simulink model "ALL_JP360_DBW_V6_5_1103"  (R2022a)
settings: Solver=FixedStepAuto  StartTime=0.0  StopTime=inf  FixedStep=0.01  RelTol=1e-3  EnableMultiTasking=on
model workspace (MAT data in the model file):
  g = 9.8
undefined symbols (not defined in the file or in its folder): canChannel, delta_v_p, IPM_Line_C0, IPM_Line_C1, IPM_Line_C2, IPM_Line_C3, M, M_p, MRR_ObjDistX, MRR_ObjDistY, MRR_ObjFusionCamID, MRR_ObjFusionSig, MRR_ObjID, MRR_ObjRelVelX, MRR_ObjRelVelY, MRR_ObjType, MRR_ObjUpdFlg, none, obj_vaild, untracktime, V, videoinput
libraries: canfdmsglib x230, canfdlib x76, slpidlib x24, simulink x18, dspstat3 x14, ctrlSharedLib x1, simulink_extras x1, imaqlib x1, realtime_pacer_lib x1, dspvision x1, visionsinks x1
(part 8 of 55)

== system ALL_JP360_DBW_V6_5_1103/MsgToCAN/CCAN_ADCU_MsgFromCAN ==
  ACC_Torque_Request : Inport
  ACC_Torque_Request_Status : Inport  Port=2
  ACC_TgtAx : Inport  Port=3
  ACC_BrakePreferred : Inport  Port=4
  ACC_StandstillReq : Inport  Port=5
  ACC_Status : Inport  Port=6
  setvspped : Inport  Port=7
  ACC_TimeGapSet : Inport  Port=8
  ACC_EngineStartstop : Inport  Port=9
  IPM_LaneAssit_Status : Inport  Port=10
  IPM_LaneAssit_TorqueReq : Inport  Port=11
  IPM_LaneAssit_TorqueReqStatus : Inport  Port=12
  Obj_Speed : Inport  Port=13
  ACC_ObjDetected : Inport  Port=14
  MRR_L_Obj_0x_class : Inport  Port=15
  MRR_L_Object_dx : Inport  Port=16
  MRR_L_Object_dy : Inport  Port=17
  MRR_LeftTargetDetection : Inport  Port=18
  MRR_R_Obj_0x_class : Inport  Port=19
  MRR_R_Object_dx : Inport  Port=20
  MRR_R_Object_dy : Inport  Port=21
  MRR_RightTargetDetection : Inport  Port=22
  MRR_F_Object_dx : Inport  Port=23
  MRR_F_Object_dy : Inport  Port=24
  MRR_F_Obj_0x_class : Inport  Port=25
  640 : Inport  Port=26
  641 : Inport  Port=27
  642 : Inport  Port=28
  643 : Inport  Port=29
  ACC_DriveOff : Inport  Port=30
  Add : Sum  Inputs=+-
  Bus Selector : BusSelector  OutputSignals=IPM_Line01_Existence_Probability,IPM_Line01_ColorClass,IPM_Line01_Type
  Bus Selector1 : BusSelector  OutputSignals=IPM_Line02_Existence_Probability,IPM_Line02_Type,IPM_Line02_ColorClass
  CCAN_ADCU_ADCU_0x538 : Subsystem  Commented=on  TreatAsAtomicUnit=on
  CCAN_ADCU_ADCU_CanTSyn_0x570 : Subsystem  Commented=on  TreatAsAtomicUnit=on
  CCAN_ADCU_ADCU_DiagResp : Subsystem  Commented=on  TreatAsAtomicUnit=on
  CCAN_ADCU_IPM_0x245 : Subsystem  TreatAsAtomicUnit=on  SystemSampleTime=0.02
  CCAN_ADCU_IPM_0x247 : Subsystem  Commented=on  TreatAsAtomicUnit=on
  CCAN_ADCU_IPM_LeftLine_0x278 : Subsystem  TreatAsAtomicUnit=on
  CCAN_ADCU_IPM_LeftLine_0x280 : Subsystem  TreatAsAtomicUnit=on
  CCAN_ADCU_IPM_RightLine_0x490 : Subsystem  TreatAsAtomicUnit=on
  CCAN_ADCU_IPM_RightLine_0x491 : Subsystem  TreatAsAtomicUnit=on
  CCAN_ADCU_IPM_VLC_0x293 : Subsystem  TreatAsAtomicUnit=on  SystemSampleTime=0.02
  CCAN_ADCU_MRR_0x238 : Subsystem  TreatAsAtomicUnit=on  SystemSampleTime=0.02
  CCAN_ADCU_MRR_0x239 : Subsystem  TreatAsAtomicUnit=on  SystemSampleTime=0.02
  CCAN_ADCU_MRR_0x246 : Subsystem  TreatAsAtomicUnit=on  SystemSampleTime=0.02
  CCAN_ADCU_MRR_FRObj_0x279 : Subsystem  TreatAsAtomicUnit=on
  CCAN_ADCU_MRR_LRObj_0x480 : Subsystem  TreatAsAtomicUnit=on
  CCAN_ADCU_TIMESYNC_analy_620 : Subsystem  Commented=on  TreatAsAtomicUnit=on
  Constant : Constant  OutDataTypeStr=int8
  Constant1 : Constant  Value=0  OutDataTypeStr=boolean
  Constant5 : Constant  Value=4  OutDataTypeStr=int8
  Constant6 : Constant  Value=2  OutDataTypeStr=int8
  Constant7 : Constant  OutDataTypeStr=int8
  Product : Product
  Product1 : Product
  Switch1 : Switch  Criteria=u2 > Threshold  Threshold=0.7  SaturateOnIntegerOverflow=off  InputSameDT=off
  Switch2 : Switch  Criteria=u2 > Threshold  Threshold=0.7  SaturateOnIntegerOverflow=off  InputSameDT=off
  Switch3 : Switch  Criteria=u2 ~= 0  SaturateOnIntegerOverflow=off  InputSameDT=off
  CCAN_ADCU_ADCU_0x538FromOutData : Outport  OutDataTypeStr=Bus:CCAN_ADCU_ADCU_0x538
  CCAN_ADCU_ADCU_CanTSyn_0x570FromOutData : Outport  Port=2  OutDataTypeStr=Bus:CCAN_ADCU_ADCU_CanTSyn_0x570
  CCAN_ADCU_ADCU_DiagRespFromOutData : Outport  Port=3  OutDataTypeStr=Bus:CCAN_ADCU_ADCU_DiagResp
  CCAN_ADCU_IPM_0x245FromOutData : Outport  Port=4  OutDataTypeStr=Bus:CCAN_ADCU_IPM_0x245
  CCAN_ADCU_IPM_0x247FromOutData : Outport  Port=5  OutDataTypeStr=Bus:CCAN_ADCU_IPM_0x247
  CCAN_ADCU_IPM_LeftLine_0x278FromOutData : Outport  Port=6  OutDataTypeStr=Bus:CCAN_ADCU_IPM_LeftLine_0x278
  CCAN_ADCU_IPM_LeftLine_0x280FromOutData : Outport  Port=7  OutDataTypeStr=Bus:CCAN_ADCU_IPM_LeftLine_0x280
  CCAN_ADCU_IPM_RightLine_0x490FromOutData : Outport  Port=8  OutDataTypeStr=Bus:CCAN_ADCU_IPM_RightLine_0x490
  CCAN_ADCU_IPM_RightLine_0x491FromOutData : Outport  Port=9  OutDataTypeStr=Bus:CCAN_ADCU_IPM_RightLine_0x491
  CCAN_ADCU_IPM_VLC_0x293FromOutData : Outport  Port=10  OutDataTypeStr=Bus:CCAN_ADCU_IPM_VLC_0x293
  CCAN_ADCU_MRR_0x238FromOutData : Outport  Port=11  OutDataTypeStr=Bus:CCAN_ADCU_MRR_0x238
  CCAN_ADCU_MRR_0x239FromOutData : Outport  Port=12  OutDataTypeStr=Bus:CCAN_ADCU_MRR_0x239
  CCAN_ADCU_MRR_0x246FromOutData : Outport  Port=13  OutDataTypeStr=Bus:CCAN_ADCU_MRR_0x246
  CCAN_ADCU_MRR_FRObj_0x279FromOutData : Outport  Port=14  OutDataTypeStr=Bus:CCAN_ADCU_MRR_FRObj_0x279
  CCAN_ADCU_MRR_LRObj_0x480FromOutData : Outport  Port=15  OutDataTypeStr=Bus:CCAN_ADCU_MRR_LRObj_0x480
  CCAN_ADCU_TIMESYNC_analy_620FromOutData : Outport  Port=16  OutDataTypeStr=Bus:CCAN_ADCU_TIMESYNC_analy_620
  wires:
  CCAN_ADCU_ADCU_0x538/1(CCAN_ADCU_ADCU_0x538FromOutData) -> CCAN_ADCU_ADCU_0x538FromOutData/1
  CCAN_ADCU_ADCU_CanTSyn_0x570/1(CCAN_ADCU_ADCU_CanTSyn_0x570FromOutData) -> CCAN_ADCU_ADCU_CanTSyn_0x570FromOutData/1
  CCAN_ADCU_ADCU_DiagResp/1(CCAN_ADCU_ADCU_DiagRespFromOutData) -> CCAN_ADCU_ADCU_DiagRespFromOutData/1
  CCAN_ADCU_IPM_0x245/1(CCAN_ADCU_IPM_0x245FromOutData) -> CCAN_ADCU_IPM_0x245FromOutData/1
  CCAN_ADCU_IPM_0x247/1(CCAN_ADCU_IPM_0x247FromOutData) -> CCAN_ADCU_IPM_0x247FromOutData/1
  CCAN_ADCU_IPM_LeftLine_0x278/1(CCAN_ADCU_IPM_LeftLine_0x278FromOutData) -> CCAN_ADCU_IPM_LeftLine_0x278FromOutData/1
  CCAN_ADCU_IPM_LeftLine_0x280/1(CCAN_ADCU_IPM_LeftLine_0x280FromOutData) -> CCAN_ADCU_IPM_LeftLine_0x280FromOutData/1
  CCAN_ADCU_IPM_RightLine_0x490/1(CCAN_ADCU_IPM_RightLine_0x490FromOutData) -> CCAN_ADCU_IPM_RightLine_0x490FromOutData/1
  CCAN_ADCU_IPM_RightLine_0x491/1(CCAN_ADCU_IPM_RightLine_0x491FromOutData) -> CCAN_ADCU_IPM_RightLine_0x491FromOutData/1
  CCAN_ADCU_IPM_VLC_0x293/1(CCAN_ADCU_IPM_VLC_0x293FromOutData) -> CCAN_ADCU_IPM_VLC_0x293FromOutData/1
  CCAN_ADCU_MRR_0x238/1(CCAN_ADCU_MRR_0x238FromOutData) -> CCAN_ADCU_MRR_0x238FromOutData/1
  CCAN_ADCU_MRR_0x239/1(CCAN_ADCU_MRR_0x239FromOutData) -> CCAN_ADCU_MRR_0x239FromOutData/1
  CCAN_ADCU_MRR_0x246/1(CCAN_ADCU_MRR_0x246FromOutData) -> CCAN_ADCU_MRR_0x246FromOutData/1
  CCAN_ADCU_MRR_FRObj_0x279/1(CCAN_ADCU_MRR_FRObj_0x279FromOutData) -> CCAN_ADCU_MRR_FRObj_0x279FromOutData/1
  CCAN_ADCU_MRR_LRObj_0x480/1(CCAN_ADCU_MRR_LRObj_0x480FromOutData) -> CCAN_ADCU_MRR_LRObj_0x480FromOutData/1
  CCAN_ADCU_TIMESYNC_analy_620/1(CCAN_ADCU_TIMESYNC_analy_620FromOutData) -> CCAN_ADCU_TIMESYNC_analy_620FromOutData/1
  ACC_Torque_Request/1 -> CCAN_ADCU_IPM_VLC_0x293/1(ACC_Torque_Request)
  ACC_Torque_Request_Status/1 -> CCAN_ADCU_IPM_VLC_0x293/2(ACC_Torque_Request_Status)
  ACC_TgtAx/1 -> CCAN_ADCU_MRR_0x238/1(ACC_TgtAx)
  ACC_StandstillReq/1 -> CCAN_ADCU_MRR_0x239/3(ACC_StandstillReq)
  ACC_BrakePreferred/1 -> CCAN_ADCU_MRR_0x239/1(ACC_BrakePreferred)
  ACC_Status/1 -> CCAN_ADCU_MRR_0x246/1(ACC_Status), CCAN_ADCU_MRR_0x239/2(ACC_Status)
  ACC_EngineStartstop/1 -> CCAN_ADCU_MRR_0x246/4(ACC_EngineStartstop)
  ACC_TimeGapSet/1 -> CCAN_ADCU_MRR_0x246/3(ACC_TimeGapSet)
  setvspped/1 -> CCAN_ADCU_MRR_0x246/2(setvspped)
  IPM_LaneAssit_TorqueReqStatus/1 -> CCAN_ADCU_IPM_0x245/3(IPM_LaneAssit_TorqueReqStatus)
  IPM_LaneAssit_TorqueReq/1 -> CCAN_ADCU_IPM_0x245/2(IPM_LaneAssit_TorqueReq)
  IPM_LaneAssit_Status/1 -> CCAN_ADCU_IPM_0x245/1(IPM_LaneAssit_Status), [LKAStatus]
  Obj_Speed/1 -> CCAN_ADCU_MRR_0x246/5(Obj_Speed)
  ACC_ObjDetected/1 -> CCAN_ADCU_MRR_0x246/6(ACC_ObjDetected)
  MRR_L_Obj_0x_class/1 -> CCAN_ADCU_MRR_LRObj_0x480/1(MRR_L_Obj_0x_class)
  MRR_L_Object_dx/1 -> CCAN_ADCU_MRR_LRObj_0x480/2(MRR_L_Object_dx)
  MRR_L_Object_dy/1 -> CCAN_ADCU_MRR_LRObj_0x480/3(MRR_L_Object_dy)
  MRR_LeftTargetDetection/1 -> CCAN_ADCU_MRR_LRObj_0x480/4(MRR_LeftTargetDetection)
  MRR_R_Obj_0x_class/1 -> CCAN_ADCU_MRR_LRObj_0x480/5(MRR_R_Obj_0x_class)
  MRR_R_Object_dx/1 -> CCAN_ADCU_MRR_LRObj_0x480/6(MRR_R_Object_dx)
  MRR_R_Object_dy/1 -> CCAN_ADCU_MRR_LRObj_0x480/7(MRR_R_Object_dy)
  MRR_RightTargetDetection/1 -> CCAN_ADCU_MRR_LRObj_0x480/8(MRR_RightTargetDetection)
  MRR_F_Obj_0x_class/1 -> CCAN_ADCU_MRR_FRObj_0x279/3(MRR_F_Obj_0x_class)
  MRR_F_Object_dy/1 -> CCAN_ADCU_MRR_FRObj_0x279/2(MRR_F_Object_dy)
  MRR_F_Object_dx/1 -> CCAN_ADCU_MRR_FRObj_0x279/1(MRR_F_Object_dx)
  643/1 -> CCAN_ADCU_IPM_RightLine_0x491/3(491)
  642/1 -> CCAN_ADCU_IPM_LeftLine_0x280/3(280)
  640/1 -> Bus Selector/1, CCAN_ADCU_IPM_LeftLine_0x278/1(278)
  Bus Selector/2 -> CCAN_ADCU_IPM_LeftLine_0x280/2(In1)  "<IPM_Line01_ColorClass>"
  Bus Selector/3 -> CCAN_ADCU_IPM_LeftLine_0x280/1(In2)  "<IPM_Line01_Type>"
  641/1 -> Bus Selector1/1, CCAN_ADCU_IPM_RightLine_0x490/1(490)
  Bus Selector1/2 -> CCAN_ADCU_IPM_RightLine_0x491/2(In1)  "<IPM_Line02_Type>"
  Bus Selector1/3 -> CCAN_ADCU_IPM_RightLine_0x491/1(In2)  "<IPM_Line02_ColorClass>"
  Bus Selector/1 -> [line01]  "<IPM_Line01_Existence_Probability>"
  Bus Selector1/1 -> [line02]  "<IPM_Line02_Existence_Probability>"
  Product/1 -> CCAN_ADCU_IPM_0x245/4(line01)
  Product1/1 -> CCAN_ADCU_IPM_0x245/5(line02)
  ACC_DriveOff/1 -> CCAN_ADCU_MRR_0x239/4(ACC_DriveOff)
  [line02] -> Switch2/2
  Switch1/1 -> Product/1
  Constant/1 -> Switch2/1, Switch1/1
  Switch2/1 -> Product1/1
  [line01] -> Switch1/2
  Add/1 -> Switch3/2
  Constant7/1 -> Switch3/1
  Constant5/1 -> Add/2
  [LKAStatus] -> Add/1
  Constant6/1 -> Switch3/3
  Constant1/1 -> Switch1/3, Switch2/3
  Switch3/1 -> Product/2, Product1/2

== system ALL_JP360_DBW_V6_5_1103/MsgToCAN/CCAN_ADCU_MsgToCAN ==
  CCAN_ADCU_ADCU_0x538ToInData : Inport  OutDataTypeStr=Bus:CCAN_ADCU_ADCU_0x538
  CCAN_ADCU_ADCU_CanTSyn_0x570ToInData : Inport  Port=2  OutDataTypeStr=Bus:CCAN_ADCU_ADCU_CanTSyn_0x570
  CCAN_ADCU_ADCU_DiagRespToInData : Inport  Port=3  OutDataTypeStr=Bus:CCAN_ADCU_ADCU_DiagResp
  CCAN_ADCU_IPM_0x245ToInData : Inport  Port=4  OutDataTypeStr=Bus:CCAN_ADCU_IPM_0x245
  CCAN_ADCU_IPM_0x247ToInData : Inport  Port=5  OutDataTypeStr=Bus:CCAN_ADCU_IPM_0x247
  CCAN_ADCU_IPM_LeftLine_0x278ToInData : Inport  Port=6  OutDataTypeStr=Bus:CCAN_ADCU_IPM_LeftLine_0x278
  CCAN_ADCU_IPM_LeftLine_0x280ToInData : Inport  Port=7  OutDataTypeStr=Bus:CCAN_ADCU_IPM_LeftLine_0x280
  CCAN_ADCU_IPM_RightLine_0x490ToInData : Inport  Port=8  OutDataTypeStr=Bus:CCAN_ADCU_IPM_RightLine_0x490
  CCAN_ADCU_IPM_RightLine_0x491ToInData : Inport  Port=9  OutDataTypeStr=Bus:CCAN_ADCU_IPM_RightLine_0x491
  CCAN_ADCU_IPM_VLC_0x293ToInData : Inport  Port=10  OutDataTypeStr=Bus:CCAN_ADCU_IPM_VLC_0x293
  CCAN_ADCU_MRR_0x238ToInData : Inport  Port=11  OutDataTypeStr=Bus:CCAN_ADCU_MRR_0x238
  CCAN_ADCU_MRR_0x239ToInData : Inport  Port=12  OutDataTypeStr=Bus:CCAN_ADCU_MRR_0x239
  CCAN_ADCU_MRR_0x246ToInData : Inport  Port=13  OutDataTypeStr=Bus:CCAN_ADCU_MRR_0x246
  CCAN_ADCU_MRR_FRObj_0x279ToInData : Inport  Port=14  OutDataTypeStr=Bus:CCAN_ADCU_MRR_FRObj_0x279
  CCAN_ADCU_MRR_LRObj_0x480ToInData : Inport  Port=15  OutDataTypeStr=Bus:CCAN_ADCU_MRR_LRObj_0x480
  CCAN_ADCU_TIMESYNC_analy_620ToInData : Inport  Port=16  OutDataTypeStr=Bus:CCAN_ADCU_TIMESYNC_analy_620
  CCAN_ADCU_ADCU_0x538 : Subsystem  TreatAsAtomicUnit=on
  CCAN_ADCU_ADCU_CanTSyn_0x570 : Subsystem  TreatAsAtomicUnit=on
  CCAN_ADCU_ADCU_DiagResp : Subsystem  TreatAsAtomicUnit=on
  CCAN_ADCU_IPM_0x245 : Subsystem  TreatAsAtomicUnit=on
  CCAN_ADCU_IPM_0x247 : Subsystem  TreatAsAtomicUnit=on
  CCAN_ADCU_IPM_LeftLine_0x278 : Subsystem  TreatAsAtomicUnit=on
  CCAN_ADCU_IPM_LeftLine_0x280 : Subsystem  TreatAsAtomicUnit=on
  CCAN_ADCU_IPM_RightLine_0x490 : Subsystem  TreatAsAtomicUnit=on
  CCAN_ADCU_IPM_RightLine_0x491 : Subsystem  TreatAsAtomicUnit=on
  CCAN_ADCU_IPM_VLC_0x293 : Subsystem  TreatAsAtomicUnit=on
  CCAN_ADCU_MRR_0x238 : Subsystem  TreatAsAtomicUnit=on
  CCAN_ADCU_MRR_0x239 : Subsystem  TreatAsAtomicUnit=on
  CCAN_ADCU_MRR_0x246 : Subsystem  TreatAsAtomicUnit=on
  CCAN_ADCU_MRR_FRObj_0x279 : Subsystem  TreatAsAtomicUnit=on
  CCAN_ADCU_MRR_LRObj_0x480 : Subsystem  TreatAsAtomicUnit=on
  CCAN_ADCU_TIMESYNC_analy_620 : Subsystem  TreatAsAtomicUnit=on
  CCAN_ADCU_ADCU_0x538ToOutData : Outport  OutDataTypeStr=Bus:CAN_FD_MESSAGE_BUS
  CCAN_ADCU_ADCU_CanTSyn_0x570ToOutData : Outport  Port=2  OutDataTypeStr=Bus:CAN_FD_MESSAGE_BUS
  CCAN_ADCU_ADCU_DiagRespToOutData : Outport  Port=3  OutDataTypeStr=Bus:CAN_FD_MESSAGE_BUS
  CCAN_ADCU_IPM_0x245ToOutData : Outport  Port=4  OutDataTypeStr=Bus:CAN_FD_MESSAGE_BUS
  CCAN_ADCU_IPM_0x247ToOutData : Outport  Port=5  OutDataTypeStr=Bus:CAN_FD_MESSAGE_BUS
  CCAN_ADCU_IPM_LeftLine_0x278ToOutData : Outport  Port=6  OutDataTypeStr=Bus:CAN_FD_MESSAGE_BUS
  CCAN_ADCU_IPM_LeftLine_0x280ToOutData : Outport  Port=7  OutDataTypeStr=Bus:CAN_FD_MESSAGE_BUS
  CCAN_ADCU_IPM_RightLine_0x490ToOutData : Outport  Port=8  OutDataTypeStr=Bus:CAN_FD_MESSAGE_BUS
  CCAN_ADCU_IPM_RightLine_0x491ToOutData : Outport  Port=9  OutDataTypeStr=Bus:CAN_FD_MESSAGE_BUS
  CCAN_ADCU_IPM_VLC_0x293ToOutData : Outport  Port=10  OutDataTypeStr=Bus:CAN_FD_MESSAGE_BUS
  CCAN_ADCU_MRR_0x238ToOutData : Outport  Port=11  OutDataTypeStr=Bus:CAN_FD_MESSAGE_BUS
  CCAN_ADCU_MRR_0x239ToOutData : Outport  Port=12  OutDataTypeStr=Bus:CAN_FD_MESSAGE_BUS
  CCAN_ADCU_MRR_0x246ToOutData : Outport  Port=13  OutDataTypeStr=Bus:CAN_FD_MESSAGE_BUS
  CCAN_ADCU_MRR_FRObj_0x279ToOutData : Outport  Port=14  OutDataTypeStr=Bus:CAN_FD_MESSAGE_BUS
  CCAN_ADCU_MRR_LRObj_0x480ToOutData : Outport  Port=15  OutDataTypeStr=Bus:CAN_FD_MESSAGE_BUS
  CCAN_ADCU_TIMESYNC_analy_620ToOutData : Outport  Port=16  OutDataTypeStr=Bus:CAN_FD_MESSAGE_BUS
  wires:
  CCAN_ADCU_ADCU_0x538ToInData/1 -> CCAN_ADCU_ADCU_0x538/1(CCAN_ADCU_ADCU_0x538ToInData)  "CCAN_ADCU_ADCU_0x538ToInData"
  CCAN_ADCU_ADCU_0x538/1(CCAN_ADCU_ADCU_0x538ToOutData) -> CCAN_ADCU_ADCU_0x538ToOutData/1  "CCAN_ADCU_ADCU_0x538ToOutData"
  CCAN_ADCU_ADCU_CanTSyn_0x570ToInData/1 -> CCAN_ADCU_ADCU_CanTSyn_0x570/1(CCAN_ADCU_ADCU_CanTSyn_0x570ToInData)  "CCAN_ADCU_ADCU_CanTSyn_0x570ToInData"
  CCAN_ADCU_ADCU_CanTSyn_0x570/1(CCAN_ADCU_ADCU_CanTSyn_0x570ToOutData) -> CCAN_ADCU_ADCU_CanTSyn_0x570ToOutData/1  "CCAN_ADCU_ADCU_CanTSyn_0x570ToOutData"
  CCAN_ADCU_ADCU_DiagRespToInData/1 -> CCAN_ADCU_ADCU_DiagResp/1(CCAN_ADCU_ADCU_DiagRespToInData)  "CCAN_ADCU_ADCU_DiagRespToInData"
  CCAN_ADCU_ADCU_DiagResp/1(CCAN_ADCU_ADCU_DiagRespToOutData) -> CCAN_ADCU_ADCU_DiagRespToOutData/1  "CCAN_ADCU_ADCU_DiagRespToOutData"
  CCAN_ADCU_IPM_0x245ToInData/1 -> CCAN_ADCU_IPM_0x245/1(CCAN_ADCU_IPM_0x245ToInData)  "CCAN_ADCU_IPM_0x245ToInData"
  CCAN_ADCU_IPM_0x245/1(CCAN_ADCU_IPM_0x245ToOutData) -> CCAN_ADCU_IPM_0x245ToOutData/1  "CCAN_ADCU_IPM_0x245ToOutData"
  CCAN_ADCU_IPM_0x247ToInData/1 -> CCAN_ADCU_IPM_0x247/1(CCAN_ADCU_IPM_0x247ToInData)  "CCAN_ADCU_IPM_0x247ToInData"
  CCAN_ADCU_IPM_0x247/1(CCAN_ADCU_IPM_0x247ToOutData) -> CCAN_ADCU_IPM_0x247ToOutData/1  "CCAN_ADCU_IPM_0x247ToOutData"
  CCAN_ADCU_IPM_LeftLine_0x278ToInData/1 -> CCAN_ADCU_IPM_LeftLine_0x278/1(CCAN_ADCU_IPM_LeftLine_0x278ToInData)  "CCAN_ADCU_IPM_LeftLine_0x278ToInData"
  CCAN_ADCU_IPM_LeftLine_0x278/1(CCAN_ADCU_IPM_LeftLine_0x278ToOutData) -> CCAN_ADCU_IPM_LeftLine_0x278ToOutData/1  "CCAN_ADCU_IPM_LeftLine_0x278ToOutData"
  CCAN_ADCU_IPM_LeftLine_0x280ToInData/1 -> CCAN_ADCU_IPM_LeftLine_0x280/1(CCAN_ADCU_IPM_LeftLine_0x280ToInData)  "CCAN_ADCU_IPM_LeftLine_0x280ToInData"
  CCAN_ADCU_IPM_LeftLine_0x280/1(CCAN_ADCU_IPM_LeftLine_0x280ToOutData) -> CCAN_ADCU_IPM_LeftLine_0x280ToOutData/1  "CCAN_ADCU_IPM_LeftLine_0x280ToOutData"
  CCAN_ADCU_IPM_RightLine_0x490ToInData/1 -> CCAN_ADCU_IPM_RightLine_0x490/1(CCAN_ADCU_IPM_RightLine_0x490ToInData)  "CCAN_ADCU_IPM_RightLine_0x490ToInData"
  CCAN_ADCU_IPM_RightLine_0x490/1(CCAN_ADCU_IPM_RightLine_0x490ToOutData) -> CCAN_ADCU_IPM_RightLine_0x490ToOutData/1  "CCAN_ADCU_IPM_RightLine_0x490ToOutData"
  CCAN_ADCU_IPM_RightLine_0x491ToInData/1 -> CCAN_ADCU_IPM_RightLine_0x491/1(CCAN_ADCU_IPM_RightLine_0x491ToInData)  "CCAN_ADCU_IPM_RightLine_0x491ToInData"
  CCAN_ADCU_IPM_RightLine_0x491/1(CCAN_ADCU_IPM_RightLine_0x491ToOutData) -> CCAN_ADCU_IPM_RightLine_0x491ToOutData/1  "CCAN_ADCU_IPM_RightLine_0x491ToOutData"
  CCAN_ADCU_IPM_VLC_0x293ToInData/1 -> CCAN_ADCU_IPM_VLC_0x293/1(CCAN_ADCU_IPM_VLC_0x293ToInData)  "CCAN_ADCU_IPM_VLC_0x293ToInData"
  CCAN_ADCU_IPM_VLC_0x293/1(CCAN_ADCU_IPM_VLC_0x293ToOutData) -> CCAN_ADCU_IPM_VLC_0x293ToOutData/1  "CCAN_ADCU_IPM_VLC_0x293ToOutData"
  CCAN_ADCU_MRR_0x238ToInData/1 -> CCAN_ADCU_MRR_0x238/1(CCAN_ADCU_MRR_0x238ToInData)  "CCAN_ADCU_MRR_0x238ToInData"
  CCAN_ADCU_MRR_0x238/1(CCAN_ADCU_MRR_0x238ToOutData) -> CCAN_ADCU_MRR_0x238ToOutData/1  "CCAN_ADCU_MRR_0x238ToOutData"
  CCAN_ADCU_MRR_0x239ToInData/1 -> CCAN_ADCU_MRR_0x239/1(CCAN_ADCU_MRR_0x239ToInData)  "CCAN_ADCU_MRR_0x239ToInData"
  CCAN_ADCU_MRR_0x239/1(CCAN_ADCU_MRR_0x239ToOutData) -> CCAN_ADCU_MRR_0x239ToOutData/1  "CCAN_ADCU_MRR_0x239ToOutData"
  CCAN_ADCU_MRR_0x246ToInData/1 -> CCAN_ADCU_MRR_0x246/1(CCAN_ADCU_MRR_0x246ToInData)  "CCAN_ADCU_MRR_0x246ToInData"
  CCAN_ADCU_MRR_0x246/1(CCAN_ADCU_MRR_0x246ToOutData) -> CCAN_ADCU_MRR_0x246ToOutData/1  "CCAN_ADCU_MRR_0x246ToOutData"
  CCAN_ADCU_MRR_FRObj_0x279ToInData/1 -> CCAN_ADCU_MRR_FRObj_0x279/1(CCAN_ADCU_MRR_FRObj_0x279ToInData)  "CCAN_ADCU_MRR_FRObj_0x279ToInData"
  CCAN_ADCU_MRR_FRObj_0x279/1(CCAN_ADCU_MRR_FRObj_0x279ToOutData) -> CCAN_ADCU_MRR_FRObj_0x279ToOutData/1  "CCAN_ADCU_MRR_FRObj_0x279ToOutData"
  CCAN_ADCU_MRR_LRObj_0x480ToInData/1 -> CCAN_ADCU_MRR_LRObj_0x480/1(CCAN_ADCU_MRR_LRObj_0x480ToInData)  "CCAN_ADCU_MRR_LRObj_0x480ToInData"
  CCAN_ADCU_MRR_LRObj_0x480/1(CCAN_ADCU_MRR_LRObj_0x480ToOutData) -> CCAN_ADCU_MRR_LRObj_0x480ToOutData/1  "CCAN_ADCU_MRR_LRObj_0x480ToOutData"
  CCAN_ADCU_TIMESYNC_analy_620ToInData/1 -> CCAN_ADCU_TIMESYNC_analy_620/1(CCAN_ADCU_TIMESYNC_analy_620ToInData)  "CCAN_ADCU_TIMESYNC_analy_620ToInData"
  CCAN_ADCU_TIMESYNC_analy_620/1(CCAN_ADCU_TIMESYNC_analy_620ToOutData) -> CCAN_ADCU_TIMESYNC_analy_620ToOutData/1  "CCAN_ADCU_TIMESYNC_analy_620ToOutData"

== system ALL_JP360_DBW_V6_5_1103/button/ACCset ==
  note: 0: OFF
      | 1: Passive
      | 2: Stand-By
      | 3: Active-Control
      | 5: Override
      | 6: Standstill
      | 7: Failure
  SWM_ACCSwitch : Inport
  acc_status : Inport  Port=2  OutDataTypeStr=int8
  set_speed_out : Inport  Port=3
  TimeGapSet : Inport  Port=4
  SWM_ACCvSetPlus : Inport  Port=5
  SWM_ACCvSetMinus : Inport  Port=6
  ACC_button : Subsystem
  Chart1 : Stateflow chart  TreatAsAtomicUnit=on
  accsetv4 : Stateflow chart  TreatAsAtomicUnit=on
      settings: RTWSystemCode=Reusable function
  setvspeed : Outport
  TimeGapSetOut : Outport  Port=2
  Out3 : Outport  Port=3
  wires:
  TimeGapSet/1 -> Chart1/Trigger
  SWM_ACCSwitch/1 -> [SWM_ACCSwitch]
  SWM_ACCvSetPlus/1 -> [SWM_ACCvSetPlus]
  SWM_ACCvSetMinus/1 -> [SWM_ACCvSetMinus]
  Chart1/1(TimeGapSet) -> accsetv4/2(speed)
  [accsinp] -> accsetv4/1(accs)
  accsetv4/1(speedout) -> TimeGapSetOut/1
  ACC_button/1(setvspeed) -> setvspeed/1
  acc_status/1 -> ACC_button/1(Input), [accsinp]
  [SWM_ACCvSetMinus] -> ACC_button/4(SWM_ACCvSetMinus)
  [SWM_ACCvSetPlus] -> ACC_button/3(SWM_ACCvSetPlus)
  [SWM_ACCSwitch] -> ACC_button/2(SWM_ACCSwitch)
  ACC_button/2(SWM_ACCSwitchOut) -> Out3/1
  set_speed_out/1 -> ACC_button/5(set_speed_out)

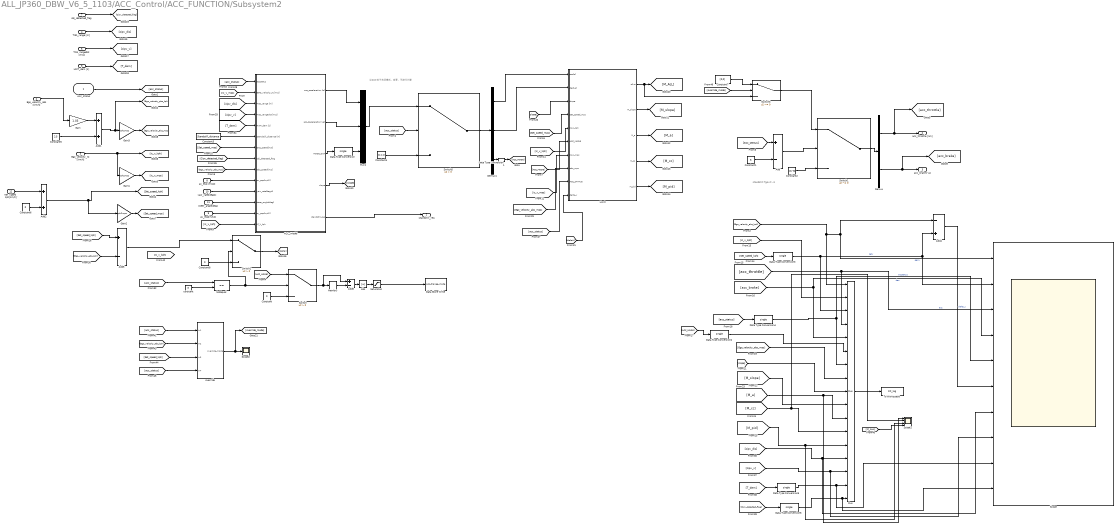
== system ALL_JP360_DBW_V6_5_1103/ACC_Control/ACC_FUNCTION/Subsystem2 ==
  note: standstill
      | TgAx= -3
  note: 当ACC处于关闭模式，发零，不进行计算
  Acc_status : Inport
  Ego_velocity_abs [km/h] : Inport  Port=2
  Ego_velocity_IC [km/h] : Inport  Port=3
  TIS1_range [m] : Inport  Port=4
  TIS1_rangedot [m/s] : Inport  Port=5
  HWT_dem [s] : Inport  Port=6
  obj_detacted_flag : Inport  Port=7
  ax_esp [m/s2] : Inport  Port=8
  ay_esp[m/s2] : Inport  Port=9
  yaw_rate[deg/s] : Inport  Port=10
  steer_angle[deg] : Inport  Port=11
  Set_speed_kph[km/h] : Inport  Port=12
  ACC_model : Subsystem
  Abs : Abs  SaturateOnIntegerOverflow=off
  Add : Sum  Inputs=+-
  Add1 : Sum
  Add2 : Sum
  Add4 : Sum  Inputs=-+
  Add5 : Sum  Inputs=+-
  Add6 : Sum  Inputs=+-
  Constant : Constant  Value=0  OutDataTypeStr=single
  Constant1 : Constant  Value=6  OutDataTypeStr=int8
  Constant2 : Constant  Value=[0,-3]  OutDataTypeStr=single
  Constant3 : Constant  Value=Standstill_distance  OutDataTypeStr=single
  Constant4 : Constant  Value=[0,0,0]  OutDataTypeStr=single
  Constant5 : Constant  Value=2.5  OutDataTypeStr=single
  Constant6 : Constant  Value=0  OutDataTypeStr=single
  Constant7 : Constant  Value=[0,0]  OutDataTypeStr=single
  Constant8 : Constant  Value=0  OutDataTypeStr=single
  Data Store Write : DataStoreWrite  DataStoreName=acc_change_mode  IndexOptions=Index vector (dialog)  Indices=1  OutputSizes=1
  Data Type Conversion{,2..6} (6 alike) : DataTypeConversion  OutDataTypeStr=single  SaturateOnIntegerOverflow=off  RndMeth=Floor
  Data Type Conversion1 : DataTypeConversion  OutDataTypeStr=int8  SaturateOnIntegerOverflow=off  RndMeth=Floor
  Demux : Demux  Outputs=2
  Demux1 : Demux  Outputs=3
  Gain : Gain  Gain=1.03
  Gain1 : Gain  Gain=kph2mps
  Gain2 : Gain  Gain=kph2mps
  Gain3 : Gain  Gain=kph2mps
  Limit : Subsystem  mask{V_limit_line=70, Uplimit_a=1.8, Lowlimit_a=1.5, Dec_dead_zone=0.05, Dec_Drag=0.1, Dec_limit_line=-0.6, Delta_dec_uplimit=0.13, Delta_dec_lowlimit0=-0.08, Delta_dec_lowlimit1=-0.08}
      mask prompts: V_limit_line "速度阈值V_limit_line"; Uplimit_a "速度大于阈值时限制加速度Uplimit_a"; Lowlimit_a "速度小于阈值时限制加速度Lowlimit_a"; Dec_dead_zone "减速度死区Dec_dead_zone"; Dec_Drag "减速度请求EMS反拖扭矩Dec_Drag"; Dec_limit_line "减速度阈值Dec_limit_line"; Delta_dec_uplimit "减速度上升斜率限制Delta_dec_uplimit"; Delta_dec_lowlimit0 "减速度下降斜率限制Delta_dec_lowlimit0"; Delta_dec_lowlimit1 "减速度下降斜率限制Delta_dec_lowlimit1"
      mask DialogControl ParameterGroupVar Prompt: 参数
  Memory : Memory
  Mux : Mux  Inputs=17
  Mux1 : Mux  Inputs=3
  NotEqual : RelationalOperator  Operator===  OutDataTypeStr=boolean  RndMeth=Simplest  InputSameDT=off
  Saturation : Saturate  UpperLimit=1  LowerLimit=0
  Scope : Scope  NumInputPorts=10
  Scope1 : Scope  NumInputPorts=4
  Scope2 : Scope
  Switch : Switch  Criteria=u2 > Threshold  SaturateOnIntegerOverflow=off  InputSameDT=off
  Switch1 : Switch  Criteria=u2 ~= 0  SaturateOnIntegerOverflow=off  InputSameDT=off
  Switch2 : Switch  Criteria=u2 > Threshold  SaturateOnIntegerOverflow=off  InputSameDT=off
  Switch3 : Switch  Criteria=u2 ~= 0  SaturateOnIntegerOverflow=off  InputSameDT=off
  Switch5 : Switch  Criteria=u2 > Threshold  SaturateOnIntegerOverflow=off  InputSameDT=off
  To Workspace : ToWorkspace  VariableName=CC_log  SaveFormat=Timeseries  SampleTime=-1
  constant : Constant  Value=3  OutDataTypeStr=int8  SampleTime=0.04
  override : Subsystem
  standstill_req : Outport  InitialOutput=[150]
  acc_throttle [nm] : Outport  Port=2
  acc_brake [-a] : Outport  Port=3
  wires:
  Limit/3(M_a) -> [M_a]
  Limit/2(M_slope) -> [M_slope]
  Limit/5(M_pid) -> [M_pid]
  Limit/4(M_cc) -> [M_cc]
  [slope] -> Limit/3(slope)
  ACC_model/4(slope) -> [slope]
  [Ic_v_mps] -> Limit/7(IC_V_mps)
  [Ic_v_kph] -> Limit/5(IC_V_kph)
  [Ic_v_mps] -> ACC_model/2(EGO_velocity_IC [m/s])
  Gain3/1 -> [Ego_velocity_abs_mps]
  Gain2/1 -> [Set_speed_mps]
  Gain1/1 -> [Ic_v_mps]
  Ego_velocity_IC [km/h]/1 -> [Ic_v_kph], Gain1/1
  [Set_speed_mps] -> ACC_model/7(Des_speed[m/s])
  Data Type Conversion1/1 -> [ACC_MODE]
  [ACC_MODE] -> Limit/6(ACC_MODE)
  Data Type Conversion/1 -> Mux1/3
  [Ic_v_kph] -> ACC_model/14(IC_V_kph)
  [Set_speed_mps] -> Limit/4(Set_speed_mps)
  ay_esp[m/s2]/1 -> ACC_model/13(ay_esp[m/s2])
  steer_angle[deg]/1 -> ACC_model/12(steer_angle[deg])
  yaw_rate[deg/s]/1 -> ACC_model/11(yaw_rate[deg/s])
  ax_esp [m/s2]/1 -> ACC_model/10(ax_esp[m/s2])
  [Ego_velocity_abs_mps] -> ACC_model/9(abs_speed[m/s])
  Constant3/1 -> ACC_model/6(Standstill_distance [m])
  Acc_status/1 -> [acc_status]
  [acc_status] -> Add/1
  Limit/1(a&-a) -> Switch3/3, [M_ALL]
  Add/1 -> Switch1/2
  Constant1/1 -> Add/2
  Constant2/1 -> Switch1/3
  Switch1/1 -> Demux/1
  Demux1/2 -> Limit/2(dec[-a])
  Demux1/1 -> Limit/1(acc[a])
  Mux1/1 -> Switch5/1
  ACC_model/3(MODE_OUT) -> Data Type Conversion/1
  ACC_model/2(acc_deceleration [-a]) -> Mux1/2
  ACC_model/1(acc_acceleration [a]) -> Mux1/1
  Demux1/3 -> Data Type Conversion1/1
  [acc_status] -> Switch5/2
  Switch5/1 -> Demux1/1
  Constant4/1 -> Switch5/3
  Ego_velocity_abs [km/h]/1 -> Gain/1
  Demux/2 -> acc_brake [-a]/1, [acc_brake]
  Demux/1 -> acc_throttle [nm]/1, [acc_throttle]
  ACC_model/5(standstill_req) -> standstill_req/1
  [acc_status] -> NotEqual/1
  Constant/1 -> Switch/3
  constant/1 -> NotEqual/2
  Add6/1 -> Abs/1
  NotEqual/1 -> Switch2/2, Switch/2
  [ACC_MODE] -> Switch/1
  [acc_status] -> Data Type Conversion4/1
  [Set_speed_kph] -> Data Type Conversion3/1
  [ACC_MODE] -> Data Type Conversion2/1
  Data Type Conversion4/1 -> Scope/5, Mux/7  "accstatus"
  Data Type Conversion2/1 -> Mux/6
  [Ego_velocity_abs_mps] -> Mux/8
  Data Type Conversion3/1 -> Add4/2, Scope/2, Mux/3  "setv"
  [acc_brake] -> Scope/4, Mux/5  "dec"
  [acc_throttle] -> Scope/3, Mux/4  "acc"
  [M_slope] -> Mux/10
  [M_a] -> Scope1/1, Mux/11
  [slope] -> Mux/9
  [M_cc] -> Scope1/2, Mux/12
  [Ic_v_kph] -> Mux/2
  [M_pid] -> Scope1/3, Mux/13
  [Ego_velocity_abs_kph] -> Mux/1, Add4/1, Scope/1  "egov"
  Mux/1 -> To Workspace/1
  [Ego_velocity_abs_mps] -> Limit/8(abs_mps)
  [acc_status] -> Limit/9(ACC_STATUS)
  [acc_status] -> ACC_model/1(accstatus)
  Gain/1 -> Add1/1
  Constant5/1 -> Add1/2
  Add1/1 -> [Ego_velocity_abs_kph], Gain3/1
  Add2/1 -> Gain2/1, [Set_speed_kph]
  Set_speed_kph[km/h]/1 -> Add2/1
  Constant6/1 -> Add2/2
  Add4/1 -> Scope/6  "delta_v"
  [Set_speed_kph] -> Add5/1
  [Ego_velocity_abs_kph] -> Add5/2
  Add5/1 -> Switch2/1
  [deltaV] -> Limit/10(delta_v)
  Switch2/1 -> [deltaV]
  Constant8/1 -> Switch2/3
  TIS1_range [m]/1 -> [cipv_dis]
  TIS1_rangedot [m/s]/1 -> [cipv_v]
  HWT_dem [s]/1 -> [T_dem]
  [cipv_dis] -> ACC_model/3(TIS1_range [m])
  [cipv_v] -> ACC_model/4(TIS1_rangedot [m/s])
  [T_dem] -> ACC_model/5(HWT_dem [s])
  obj_detacted_flag/1 -> [Cipv_detected_flag]
  [Cipv_detected_flag] -> ACC_model/8(obj_detacted_flag)
  [T_dem] -> Data Type Conversion5/1
  [cipv_v] -> Scope/8, Mux/15
  [Cipv_detected_flag] -> Data Type Conversion6/1
  [cipv_dis] -> Scope/7, Mux/14
  Data Type Conversion5/1 -> Scope/9, Mux/16
  Data Type Conversion6/1 -> Scope/10, Mux/17
  [M_ALL] -> Scope1/4
  Switch/1 -> Add6/1, Memory/1
  Memory/1 -> Add6/2
  Abs/1 -> Saturation/1
  [acc_status] -> override/1(In1)
  [Ego_velocity_abs_kph] -> override/2(In2)
  [Set_speed_kph] -> override/3(In3)
  [acc_status] -> override/4(In4)
  override/1(override_mode) -> [override_mode], Scope2/1
  [override_mode] -> Switch3/2
  Switch3/1 -> Switch1/1
  Constant7/1 -> Switch3/1
  Saturation/1 -> Data Store Write/1

== system ALL_JP360_DBW_V6_5_1103/ACC_Control/ACC_FUNCTION/acc_stateflow ==
  SWM_ACCSwitch : Inport
  SWM_ACCSet : Inport  Port=2
  SWM_ACCResume : Inport  Port=3
  BCM_DoorStsFrntLe : Inport  Port=4
  BCM_DoorStsFrntRi : Inport  Port=5
  BCM_DoorStsRearLe : Inport  Port=6
  BCM_DoorStsRearRi : Inport  Port=7
  BCM_PowerModeInvalid : Inport  Port=8
  BCM_PowerMode : Inport  Port=9
  BCM_Mechanical_Hand_Brake : Inport  Port=10
  BCM_EnginehoodSts : Inport  Port=11
  IPM_SensorState : Inport  Port=12
  MRR_HWFail : Inport  Port=13
  SRS_SBR_Driver : Inport  Port=14
  EMS_IndicatedEngError : Inport  Port=15
  EMS_AccRAWPedalRatio : Inport  Port=16
  EMS_BrkPedalStasus : Inport  Port=17
  EPS_EPSPAMSts : Inport  Port=18
  TCU_GearSelectorReq : Inport  Port=19
  ESP_EPBStatus : Inport  Port=20
  ESP_EspEnableSts : Inport  Port=21
  ABS_VehSpdDirection : Inport  Port=22
  ESP_AvhActive : Inport  Port=23
  ESP_VehicleStandstill : Inport  Port=24
  acc_state_sw : Inport  Port=25
  EMS_IndicatedDriverOverride : Inport  Port=26
  ABS_VehSpdLgt : Inport  Port=27
  set_speed_in : Inport  Port=28
  ACC_ObjDetected : Inport  Port=29
  Obj_Speed : Inport  Port=30
  CIPV_ObjDistX : Inport  Port=31
  Chart2 : Stateflow chart  TreatAsAtomicUnit=on
  Chart3 : Stateflow chart  TreatAsAtomicUnit=on
  Data Type Conversion1 : DataTypeConversion  OutDataTypeStr=uint8  SaturateOnIntegerOverflow=off  RndMeth=Floor
  Delay1 : Delay  DelayLength=1
  Delay2 : Delay  DelayLength=1
  Gain : Gain  Gain=3.6
  Scope : Scope
  Scope2 : Scope  NumInputPorts=2
  ACC_Status : Outport
  set_speed_out : Outport  Port=2
  ACC_DriveOff : Outport  Port=3
  wires:
  Chart2/1(ACC_Status) -> ACC_Status/1, Delay1/1
  SWM_ACCSwitch/1 -> Chart2/1(SWM_ACCSwitch)
  SWM_ACCSet/1 -> Chart2/2(SWM_ACCSet)
  SWM_ACCResume/1 -> Chart3/1(u1), Chart2/3(SWM_ACCResume)
  BCM_DoorStsFrntLe/1 -> Chart2/4(BCM_DoorStsFrntLe)
  BCM_DoorStsFrntRi/1 -> Chart2/5(BCM_DoorStsFrntRi)
  BCM_DoorStsRearLe/1 -> Chart2/6(BCM_DoorStsRearLe)
  BCM_DoorStsRearRi/1 -> Chart2/7(BCM_DoorStsRearRi)
  BCM_PowerModeInvalid/1 -> Chart2/8(BCM_PowerModeInvalid)
  BCM_PowerMode/1 -> Chart2/9(BCM_PowerMode)
  BCM_Mechanical_Hand_Brake/1 -> Chart2/10(BCM_Mechanical_Hand_Brake)
  BCM_EnginehoodSts/1 -> Chart2/11(BCM_EnginehoodSts)
  IPM_SensorState/1 -> Chart2/12(IPM_SensorState)
  MRR_HWFail/1 -> Chart2/13(MRR_HWFail)
  SRS_SBR_Driver/1 -> Chart2/14(SRS_SBR_Driver)
  EMS_IndicatedEngError/1 -> Chart2/15(EMS_IndicatedEngError)
  EMS_BrkPedalStasus/1 -> Chart2/17(EMS_BrkPedalStasus)
  EPS_EPSPAMSts/1 -> Chart2/18(EPS_EPSPAMSts)
  TCU_GearSelectorReq/1 -> Chart2/19(TCU_GearSelectorReq)
  ESP_EPBStatus/1 -> Chart2/20(ESP_EPBStatus)
  ESP_EspEnableSts/1 -> Chart2/21(ESP_EspEnableSts)
  ABS_VehSpdDirection/1 -> Chart2/22(ABS_VehSpdDirection)
  ESP_AvhActive/1 -> Chart2/23(ESP_AvhActive)
  Chart3/1(ACC_DriveOff) -> Scope2/2, ACC_DriveOff/1, Scope/1, Chart2/25(DriveOff)
  acc_state_sw/1 -> Chart2/26(acc_state_sw)
  EMS_AccRAWPedalRatio/1 -> Chart2/16(EMS_AccRAWPedalRatio)
  ABS_VehSpdLgt/1 -> Data Type Conversion1/1
  EMS_IndicatedDriverOverride/1 -> Chart3/3(EMS_IndicatedDriverOverride), Chart2/29(EMS_IndicatedDriverOverride)
  Chart2/2(set_speed_out) -> set_speed_out/1
  Data Type Conversion1/1 -> Chart2/28(ABS_VehSpdLgt)
  set_speed_in/1 -> Chart2/27(set_speed_in)
  Chart2/3(three_s) -> Delay2/1
  Delay2/1 -> Chart3/6(three_s)
  Delay1/1 -> Chart3/2(ACC_Status)
  ACC_ObjDetected/1 -> Chart3/4(ACC_ObjDetected)
  Obj_Speed/1 -> Gain/1
  CIPV_ObjDistX/1 -> Chart3/7(CIPV_ObjDistX)
  Gain/1 -> Chart3/5(Obj_Speed)
  ESP_VehicleStandstill/1 -> Scope2/1, Chart2/24(ESP_VehicleStandstill)

== system ALL_JP360_DBW_V6_5_1103/CIPV1/Obstacle selection/Subsystem ==
  MRR_ObjID : Inport
  MRR_ObjDistX : Inport  Port=2
  MRR_ObjDistY : Inport  Port=3
  MRR_ObjRelVelX : Inport  Port=4
  MRR_ObjRelVelY : Inport  Port=5
  MRR_ObjType : Inport  Port=6
  CIPV_index1 : Inport  Port=7  OutMin=1
  CIPV_index2 : Inport  Port=8  OutMin=1
  left_obj_idx : Inport  Port=9  OutMin=1
  right_obj_idx : Inport  Port=10  OutMin=1
  MRR_ObjUpdFlg : Inport  Port=11
  CIPV1_ObjDetected : Inport  Port=12
  CIPV2_ObjDetected : Inport  Port=13
  left_obj_vaild : Inport  Port=14
  right_obj_vaild : Inport  Port=15
  IPM_Obj : Inport  Port=16
  MRR_ObjFusionSig : Inport  Port=17
  MRR_ObjFusionCamID : Inport  Port=18
  CIPV1_ObjDetected1 : Inport  Port=19
  Subsystem : Subsystem
  Subsystem1 : Subsystem
  Subsystem2 : Subsystem
  Subsystem3 : Subsystem
  cipv1 : Outport
  cipv2 : Outport  Port=2
  left_obj : Outport  Port=3
  right_obj : Outport  Port=4
  wires:
  CIPV_index1/1 -> [CIPV_index1]
  CIPV_index2/1 -> [CIPV_index2]
  left_obj_idx/1 -> [left_obj_idx]
  right_obj_idx/1 -> [right_obj_idx]
  MRR_ObjID/1 -> [MRR_ObjID]
  MRR_ObjDistX/1 -> [MRR_ObjDistX]
  MRR_ObjDistY/1 -> [MRR_ObjDistY]
  MRR_ObjRelVelX/1 -> [MRR_ObjRelVelX]
  MRR_ObjRelVelY/1 -> [MRR_ObjRelVelY]
  MRR_ObjType/1 -> [MRR_ObjType]
  Subsystem/1(cipv1) -> cipv1/1
  [MRR_ObjID] -> Subsystem/1(MRR_ObjID)
  [MRR_ObjDistX] -> Subsystem/2(MRR_ObjDistX)
  [MRR_ObjDistY] -> Subsystem/3(MRR_ObjDistY)
  [MRR_ObjRelVelX] -> Subsystem/4(MRR_ObjRelVelX)
  [MRR_ObjRelVelY] -> Subsystem/5(MRR_ObjRelVelY)
  [MRR_ObjType] -> Subsystem/6(MRR_ObjType)
  [CIPV_index1] -> Subsystem/7(CIPV_index1)
  MRR_ObjUpdFlg/1 -> [MRR_ObjUpdFlg]
  [MRR_ObjUpdFlg] -> Subsystem/8(MRR_ObjUpdFlg)
  CIPV1_ObjDetected/1 -> Subsystem/9(obj_vaild)
  Subsystem3/1(cipv1) -> cipv2/1
  [MRR_ObjUpdFlg] -> Subsystem3/8(MRR_ObjUpdFlg)
  [MRR_ObjType] -> Subsystem3/6(MRR_ObjType)
  [MRR_ObjRelVelX] -> Subsystem3/4(MRR_ObjRelVelX)
  [MRR_ObjDistX] -> Subsystem3/2(MRR_ObjDistX)
  [MRR_ObjRelVelY] -> Subsystem3/5(MRR_ObjRelVelY)
  [CIPV_index2] -> Subsystem3/7(CIPV_index1)
  [MRR_ObjDistY] -> Subsystem3/3(MRR_ObjDistY)
  CIPV2_ObjDetected/1 -> Subsystem3/9(obj_vaild)
  [MRR_ObjID] -> Subsystem3/1(MRR_ObjID)
  left_obj_vaild/1 -> Subsystem1/9(obj_vaild)
  [MRR_ObjRelVelY] -> Subsystem1/5(MRR_ObjRelVelY)
  [MRR_ObjDistX] -> Subsystem1/2(MRR_ObjDistX)
  [MRR_ObjUpdFlg] -> Subsystem1/8(MRR_ObjUpdFlg)
  [MRR_ObjRelVelX] -> Subsystem1/4(MRR_ObjRelVelX)
  [MRR_ObjType] -> Subsystem1/6(MRR_ObjType)
  [MRR_ObjDistY] -> Subsystem1/3(MRR_ObjDistY)
  [left_obj_idx] -> Subsystem1/7(CIPV_index1)
  [MRR_ObjID] -> Subsystem1/1(MRR_ObjID)
  [MRR_ObjID] -> Subsystem2/1(MRR_ObjID)
  [MRR_ObjDistY] -> Subsystem2/3(MRR_ObjDistY)
  [MRR_ObjType] -> Subsystem2/6(MRR_ObjType)
  [MRR_ObjRelVelY] -> Subsystem2/5(MRR_ObjRelVelY)
  [right_obj_idx] -> Subsystem2/7(CIPV_index1)
  [MRR_ObjDistX] -> Subsystem2/2(MRR_ObjDistX)
  right_obj_vaild/1 -> Subsystem2/9(obj_vaild)
  [MRR_ObjRelVelX] -> Subsystem2/4(MRR_ObjRelVelX)
  Subsystem2/1(cipv1) -> right_obj/1
  [MRR_ObjUpdFlg] -> Subsystem2/8(MRR_ObjUpdFlg)
  Subsystem1/1(cipv1) -> left_obj/1
  IPM_Obj/1 -> [IPM_Obj]
  MRR_ObjFusionCamID/1 -> [MRR_ObjFusionCamID]
  MRR_ObjFusionSig/1 -> [MRR_ObjFusionSig]
  [MRR_ObjFusionSig] -> Subsystem/11(MRR_ObjFusionSig)
  [IPM_Obj] -> Subsystem/10(IPM_obj)
  [MRR_ObjFusionCamID] -> Subsystem/12(MRR_ObjFusionCamID)
  [IPM_Obj] -> Subsystem3/10(IPM_obj)
  [MRR_ObjFusionSig] -> Subsystem3/11(MRR_ObjFusionSig)
  [MRR_ObjFusionCamID] -> Subsystem3/12(MRR_ObjFusionCamID)
  [IPM_Obj] -> Subsystem1/10(IPM_obj)
  [MRR_ObjFusionSig] -> Subsystem1/11(MRR_ObjFusionSig)
  [MRR_ObjFusionCamID] -> Subsystem1/12(MRR_ObjFusionCamID)
  [IPM_Obj] -> Subsystem2/10(IPM_obj)
  [MRR_ObjFusionSig] -> Subsystem2/11(MRR_ObjFusionSig)
  [MRR_ObjFusionCamID] -> Subsystem2/12(MRR_ObjFusionCamID)

== system ALL_JP360_DBW_V6_5_1103/CIPV1/Obstacle selection/Subsystem1 ==
  now_cipv1 : Inport
  last_cipv1 : Inport  Port=2
  IPM_Obj : Inport  Port=3
  Bus Assignment1 : BusAssignment  AssignedSignals=untracktime
  Bus Selector : BusSelector  OutputSignals=obj_vaild,untracktime
  Bus Selector1 : BusSelector  OutputSignals=obj_vaild
  Bus Selector3 : BusSelector  OutputSignals=untracktime
  Constant1 : Constant  OutDataTypeStr=single
  If : If  NumInputs=3  IfExpression=u1 < 0  ElseIfExpressions=u2>10, u3>0
  If Action Subsystem : Subsystem  TreatAsAtomicUnit=on
  If Action Subsystem1 : Subsystem  TreatAsAtomicUnit=on
  If Action Subsystem2 : Subsystem  TreatAsAtomicUnit=on
  If Action Subsystem3 : Subsystem  TreatAsAtomicUnit=on
  Merge : Merge  Inputs=4
  Plus3 : Sum
  out_cipv1 : Outport
  wires:
  now_cipv1/1 -> [now_cipv1]
  If/4 -> If Action Subsystem2/Action
  Bus Selector1/1 -> If/3  "<obj_vaild>"
  If/1 -> If Action Subsystem/Action
  [now_cipv1] -> If Action Subsystem/1(In1)
  If Action Subsystem/1(Out1) -> Merge/1
  [now_cipv1] -> If Action Subsystem1/1(now_cipv1)
  [last_cipv1] -> If Action Subsystem1/2(last_cipv1)
  [last_cipv1] -> If Action Subsystem2/1(last_cipv1)
  Merge/1 -> out_cipv1/1
  [now_cipv1] -> Bus Selector1/1
  Bus Selector/1 -> If/1  "<obj_vaild>"
  Bus Selector/2 -> If/2  "<untracktime>"
  [now_cipv1] -> If Action Subsystem3/1(In1)
  If/2 -> If Action Subsystem3/Action
  If Action Subsystem1/1(Out1) -> Merge/3
  If Action Subsystem2/1(Out1) -> Merge/4
  If/3 -> If Action Subsystem1/Action
  If Action Subsystem3/1(Out1) -> Merge/2
  [last_cipv1] -> Bus Selector/1
  Plus3/1 -> Bus Assignment1/2
  last_cipv1/1 -> Bus Selector3/1, Bus Assignment1/1
  Constant1/1 -> Plus3/2
  Bus Assignment1/1 -> [last_cipv1]
  Bus Selector3/1 -> Plus3/1  "<untracktime>"
  IPM_Obj/1 -> [IPM_Obj]
  [IPM_Obj] -> If Action Subsystem2/2(IPM_Obj)

== system ALL_JP360_DBW_V6_5_1103/CIPV1/Obstacle selection/get min ==
  left_lane_obstacles : Inport
  MRR_ObjDistX : Inport  Port=2
  Constant : Constant  Value=200  OutDataTypeStr=single
  Constant1 : Constant  OutDataTypeStr=single
  Constant2 : Constant  Value=0  OutDataTypeStr=single
  Constant8 : Constant  Value=0  OutDataTypeStr=single
  Maximum : dspstat3/Maximum  operation=maximum  fcn=Value  indexBase=One  operateOver=Specified dimension  Dimension=1  InputProcessing=Columns as channels (frame based)  reset=None  roiEnable=off  roiType=Rectangles  roiPortion=Entire ROI  roiOutput=Individual statistics for each ROI  roiFlag=off  roundingMode=Floor  overflowMode=off  accumDataTypeStr=Inherit: Same as product output  accumLastDataTypeStr=Inherit: Same as product output
  Minimum : dspstat3/Minimum  operation=minimum  fcn=Value and Index  indexBase=One  operateOver=Specified dimension  Dimension=1  InputProcessing=Columns as channels (frame based)  reset=None  roiEnable=off  roiType=Rectangles  roiPortion=Entire ROI  roiOutput=Individual statistics for each ROI  roiFlag=off  roundingMode=Floor  overflowMode=off
      settings: SourceProductBaseCode=DS
  Product : Product
  Switch : Switch  Criteria=u2 > Threshold  SaturateOnIntegerOverflow=off  InputSameDT=off
  Switch1 : Switch  Criteria=u2 > Threshold  SaturateOnIntegerOverflow=off  InputSameDT=off
  Switch5 : Switch  Criteria=u2 ~= 0  SaturateOnIntegerOverflow=off  InputSameDT=off
  is_vaild : Outport
  idx : Outport  Port=2
  wires:
  left_lane_obstacles/1 -> Product/1
  Switch/1 -> Minimum/1
  Switch1/1 -> Switch5/1
  Constant8/1 -> Switch5/3
  Maximum/1 -> Switch5/2
  Switch5/1 -> is_vaild/1
  Constant1/1 -> Switch1/1
  Product/1 -> Maximum/1, Switch/2, Switch/1
  MRR_ObjDistX/1 -> Product/2
  Minimum/2 -> idx/1
  Minimum/1 -> Switch1/2
  Constant2/1 -> Switch1/3
  Constant/1 -> Switch/3

== system ALL_JP360_DBW_V6_5_1103/CIPV1/Obstacle selection/get min1 ==
  right_lane_obstacles : Inport
  MRR_ObjDistX : Inport  Port=2
  Constant : Constant  Value=200  OutDataTypeStr=single
  Constant1 : Constant  OutDataTypeStr=single
  Constant2 : Constant  Value=0  OutDataTypeStr=single
  Constant8 : Constant  Value=0  OutDataTypeStr=single
  Maximum : dspstat3/Maximum  operation=maximum  fcn=Value  indexBase=One  operateOver=Specified dimension  Dimension=1  InputProcessing=Columns as channels (frame based)  reset=None  roiEnable=off  roiType=Rectangles  roiPortion=Entire ROI  roiOutput=Individual statistics for each ROI  roiFlag=off  roundingMode=Floor  overflowMode=off  accumDataTypeStr=Inherit: Same as product output  accumLastDataTypeStr=Inherit: Same as product output
  Minimum : dspstat3/Minimum  operation=minimum  fcn=Value and Index  indexBase=One  operateOver=Specified dimension  Dimension=1  InputProcessing=Columns as channels (frame based)  reset=None  roiEnable=off  roiType=Rectangles  roiPortion=Entire ROI  roiOutput=Individual statistics for each ROI  roiFlag=off  roundingMode=Floor  overflowMode=off
      settings: SourceProductBaseCode=DS
  Product : Product
  Switch : Switch  Criteria=u2 > Threshold  SaturateOnIntegerOverflow=off  InputSameDT=off
  Switch1 : Switch  Criteria=u2 > Threshold  SaturateOnIntegerOverflow=off  InputSameDT=off
  Switch5 : Switch  Criteria=u2 ~= 0  SaturateOnIntegerOverflow=off  InputSameDT=off
  is_vaild1 : Outport
  idx1 : Outport  Port=2
  wires:
  Constant/1 -> Switch/3
  Minimum/1 -> Switch1/2
  Constant2/1 -> Switch1/3
  Minimum/2 -> idx1/1
  Maximum/1 -> Switch5/2
  Switch1/1 -> Switch5/1
  Switch/1 -> Minimum/1
  Constant8/1 -> Switch5/3
  right_lane_obstacles/1 -> Product/1
  MRR_ObjDistX/1 -> Product/2
  Switch5/1 -> is_vaild1/1
  Constant1/1 -> Switch1/1
  Product/1 -> Maximum/1, Switch/2, Switch/1

== system ALL_JP360_DBW_V6_5_1103/CIPV1/filter/Filter ROI objs ==
  last_vaild_objs : Inport
  MRR_ObjDistX : Inport  Port=2
  MRR_ObjDistY1 : Inport  Port=3
  Abs2 : Abs  SaturateOnIntegerOverflow=off
  Constant4 : Constant  Value=10  OutDataTypeStr=single
  GreaterThan : RelationalOperator  Operator=>  OutDataTypeStr=boolean  RndMeth=Simplest  InputSameDT=off
  GreaterThan1 : RelationalOperator  Operator=>  OutDataTypeStr=boolean  RndMeth=Simplest  InputSameDT=off
  LessThanOrEqual : RelationalOperator  Operator=<=  OutDataTypeStr=boolean  RndMeth=Simplest  InputSameDT=off
  LessThanOrEqual1 : RelationalOperator  Operator=<=  OutDataTypeStr=boolean  RndMeth=Simplest  InputSameDT=off
  Product : Product
  Switch{,1..3} (4 alike) : Switch  Criteria=u2 > Threshold  OutMin=[0]  OutMax=[80]  SaturateOnIntegerOverflow=off  InputSameDT=off
  x default : Constant  Value=0  OutDataTypeStr=single
  x default1 : Constant  Value=0  OutDataTypeStr=single
  x default2 : Constant  Value=0  OutDataTypeStr=single
  x max : Constant  Value=100  OutDataTypeStr=single
  x min : Constant  Value=0  OutDataTypeStr=single
  x min1 : Constant  Value=0  OutDataTypeStr=single
  y max : Constant  Value=4.5  OutDataTypeStr=single
  ROI objs : Outport
  wires:
  MRR_ObjDistX/1 -> Product/2
  last_vaild_objs/1 -> [last_vaild_objs]
  [last_vaild_objs] -> Product/1
  Product/1 -> LessThanOrEqual/1, Switch/2, Switch/1
  x min/1 -> Switch/3
  LessThanOrEqual/1 -> Switch1/2
  x max/1 -> LessThanOrEqual/2
  Switch/1 -> Switch1/1
  x default/1 -> Switch1/3
  Switch1/1 -> GreaterThan/1
  x default1/1 -> GreaterThan/2
  GreaterThan/1 -> [filter_x]
  y max/1 -> LessThanOrEqual1/2
  x min1/1 -> Switch2/3
  Switch3/1 -> LessThanOrEqual1/1
  LessThanOrEqual1/1 -> Switch2/2
  Switch2/1 -> GreaterThan1/1
  x default2/1 -> GreaterThan1/2
  GreaterThan1/1 -> ROI objs/1
  Abs2/1 -> Switch3/1
  [filter_x] -> Switch3/2
  Constant4/1 -> Switch3/3
  MRR_ObjDistY1/1 -> Abs2/1
  [filter_x] -> Switch2/1

== system ALL_JP360_DBW_V6_5_1103/CIPV1/filter/Filter low probability objs ==
  MRR_ObjExistProb : Inport
  MRR_ObjObstacleProb : Inport  Port=2
  MRR_ObjType : Inport  Port=3
  Constant : Constant  Value=4  OutDataTypeStr=single
  GreaterThanOrEqual : RelationalOperator  OutDataTypeStr=boolean  RndMeth=Simplest  InputSameDT=off
  GreaterThanOrEqual1 : RelationalOperator  OutDataTypeStr=boolean  RndMeth=Simplest  InputSameDT=off
  Product : Product
  Switch : Switch  Threshold=0.95  SaturateOnIntegerOverflow=off  InputSameDT=off
  Switch1 : Switch  Criteria=u2 > Threshold  SaturateOnIntegerOverflow=off  InputSameDT=off
  Switch2 : Switch  Criteria=u2 > Threshold  SaturateOnIntegerOverflow=off  InputSameDT=off
  range max : Constant  Value=0  OutDataTypeStr=single
  range max1 : Constant  OutDataTypeStr=single
  range max2 : Constant  Value=0  OutDataTypeStr=single
  range max3 : Constant  Value=0.8  OutDataTypeStr=single
  range max4 : Constant  Value=0  OutDataTypeStr=single
  ourtput_filtered : Outport
  wires:
  range max/1 -> Switch/3
  MRR_ObjExistProb/1 -> Switch/2
  Switch/1 -> Switch1/1
  range max1/1 -> Switch/1
  range max2/1 -> Switch1/3
  MRR_ObjObstacleProb/1 -> GreaterThanOrEqual/1
  range max3/1 -> GreaterThanOrEqual/2
  GreaterThanOrEqual/1 -> Switch1/2
  Switch1/1 -> [prob_filtered]
  [prob_filtered] -> Product/1
  MRR_ObjType/1 -> Product/2
  Product/1 -> GreaterThanOrEqual1/1
  Constant/1 -> GreaterThanOrEqual1/2
  GreaterThanOrEqual1/1 -> Switch2/2
  [prob_filtered] -> Switch2/1
  range max4/1 -> Switch2/3
  Switch2/1 -> ourtput_filtered/1

== system ALL_JP360_DBW_V6_5_1103/CIPV1/filter/filter lanes ==
  note: 过滤静态和未知状态的目标
  note: 1、Lane Line Construction：用于提供车道线给后续模块使用，包括感知的车道线和虚拟车道线
      | 输入：ipm_line 、方向盘转角、横摆角速度、车速
      | 输出：左、右、左左、右右车道线。以该格式输出：Y = C0 + C1 * X + 1/2 * C2 * X^2 + 1/6 * C3 * X^3
      | Y为距离参考点的横向距离，X为距离参考点的纵向距离
      | 单位：m
      | C0：近端Y轴坐标，Video_Line_0x_A_dy
      | C1：切线夹角θ，Video_Line_0x_A_ yawangle
      | C2：曲率，Video_Line_0x_ B_hor_curve
      | C3: 曲率变化率，BV_Lin_0x_hor_curvature_alteration
      | 2、filter ：滤掉空目标，概率低的目标，矩形ROI外的目标、相对行驶的目标、不在本车道的静止目标，
      | 并将障碍物分成自车道障碍物，左车道障碍物，右车道障碍物输出
      | 3、Obstacle selection：选取cipv和 相邻障碍物目标，防止CIPV防跳变，替换障碍物类型
  note: 过滤静态和未知状态的目标
  left_line : Inport
  right_line : Inport  Port=2
  MRR_ObjDistY : Inport  Port=3
  MRR_ObjRelVelY : Inport  Port=4
  last_vaild_objs : Inport  Port=5
  objs_width : Inport  Port=6
  MRR_ObjMovingSts : Inport  Port=7
  Bus Selector1 : BusSelector  OutputSignals=IPM_Line_C0,IPM_Line_C1,IPM_Line_C2,IPM_Line_C3
  Bus Selector10 : BusSelector  OutputSignals=IPM_Line_C0,IPM_Line_C1,IPM_Line_C2,IPM_Line_C3
  Constant : Constant  Value=3.75/4  OutDataTypeStr=single
  Constant{1..2,4..5,7,9} (6 alike) : Constant  Value=0  OutDataTypeStr=single
  Constant3 : Constant  Value=3.75/4  OutDataTypeStr=single
  Constant6 : Constant  OutDataTypeStr=single
  Constant8 : Constant  OutDataTypeStr=single
  Display{,1..7} (8 alike) : Display
  GreaterThan : RelationalOperator  Operator=>  OutDataTypeStr=boolean  RndMeth=Simplest  InputSameDT=off
  GreaterThan1 : RelationalOperator  Operator=>  OutDataTypeStr=boolean  RndMeth=Simplest  InputSameDT=off
  GreaterThanOrEqual : RelationalOperator  Operator=<  OutDataTypeStr=boolean  RndMeth=Simplest  InputSameDT=off
  GreaterThanOrEqual1 : RelationalOperator  Operator=<=  OutDataTypeStr=boolean  RndMeth=Simplest  InputSameDT=off
  LT : RelationalOperator  OutDataTypeStr=boolean  RndMeth=Simplest  InputSameDT=off
  LT1 : RelationalOperator  Operator=>  OutDataTypeStr=boolean  RndMeth=Simplest  InputSameDT=off
  Plus : Sum  Inputs=+--+
  Plus1 : Sum  Inputs=++--
  Product{,1..5} (6 alike) : Product
  Switch{,1..5} (6 alike) : Switch  Criteria=u2 > Threshold  SaturateOnIntegerOverflow=off  InputSameDT=off
  get obj line y : Subsystem  TreatAsAtomicUnit=on
  get obj line y1 : Subsystem  TreatAsAtomicUnit=on
  left_lane_obstacles : Outport
  right_lane_obstacles : Outport  Port=2
  ego_lane_obstacles : Outport  Port=3
  wires:
  left_line/1 -> Bus Selector10/1
  right_line/1 -> Bus Selector1/1
  Bus Selector10/1 -> get obj line y/1(<IPM_Line01_C0>)  "<IPM_Line_C0>"
  Bus Selector10/2 -> get obj line y/2(<IPM_Line01_C1>)  "<IPM_Line_C1>"
  Bus Selector10/3 -> get obj line y/3(<IPM_Line01_C2>)  "<IPM_Line_C2>"
  Bus Selector10/4 -> get obj line y/4(<IPM_Line01_C3>)  "<IPM_Line_C3>"
  Product/1 -> [last_vaild_objDistY]
  [last_vaild_objDistY] -> get obj line y/5(objs_y)
  last_vaild_objs/1 -> [last_vaild_objs]
  [last_vaild_objs] -> Product/1
  get obj line y/1(line_y) -> Display5/1, Plus/3  "left line y"
  Constant/1 -> Plus/4
  Plus/1 -> Display3/1, LT1/1, GreaterThanOrEqual1/1
  [last_vaild_objs] -> Switch/1
  Constant1/1 -> LT1/2, Switch/3
  [last_vaild_objs] -> Switch1/1
  Constant2/1 -> Switch1/3, GreaterThanOrEqual1/2
  Switch1/1 -> [ego_right_obstacles]
  Bus Selector1/1 -> get obj line y1/1(<IPM_Line01_C0>)  "<IPM_Line_C0>"
  Bus Selector1/2 -> get obj line y1/2(<IPM_Line01_C1>)  "<IPM_Line_C1>"
  Bus Selector1/3 -> get obj line y1/3(<IPM_Line01_C2>)  "<IPM_Line_C2>"
  Bus Selector1/4 -> get obj line y1/4(<IPM_Line01_C3>)  "<IPM_Line_C3>"
  [ego_right_obstacles] -> get obj line y1/5(objs_y)
  Constant5/1 -> GreaterThanOrEqual/2, Switch3/3
  [ego_right_obstacles] -> Switch3/1
  Constant4/1 -> LT/2, Switch2/3
  [ego_right_obstacles] -> Switch2/1
  Plus1/1 -> GreaterThanOrEqual/1, LT/1
  Constant3/1 -> Plus1/4
  get obj line y1/1(line_y) -> Display/1, Plus1/3  "right line y"
  [ego_right_vaild_objDistY] -> Display1/1, Plus1/1
  LT/1 -> Switch2/2
  GreaterThanOrEqual/1 -> Switch3/2
  [ego_right_obstacles] -> Product1/1
  Product1/1 -> [ego_right_vaild_objDistY]
  Switch2/1 -> Display2/1, ego_lane_obstacles/1
  LT1/1 -> Switch/2
  GreaterThanOrEqual1/1 -> Switch1/2
  objs_width/1 -> [objs_width]
  [objs_width] -> Product2/2
  Product2/1 -> Plus1/2
  [ego_right_obstacles] -> Product2/1
  [objs_width] -> Product3/2
  [last_vaild_objs] -> Display7/1, Product3/1
  Product3/1 -> Plus/2, Display6/1
  Switch/1 -> [left_lane_obstacles]
  MRR_ObjMovingSts/1 -> [MRR_ObjMovingSts]
  [left_lane_obstacles] -> Product4/1
  [MRR_ObjMovingSts] -> Product4/2
  Product4/1 -> GreaterThan/1
  Constant6/1 -> GreaterThan/2
  GreaterThan/1 -> Switch4/2
  [left_lane_obstacles] -> Switch4/1
  Constant7/1 -> Switch4/3
  Switch4/1 -> left_lane_obstacles/1
  Switch3/1 -> [right_lane_obstacles]
  Constant9/1 -> Switch5/3
  [MRR_ObjMovingSts] -> Product5/2
  [right_lane_obstacles] -> Product5/1
  Switch5/1 -> right_lane_obstacles/1
  Product5/1 -> GreaterThan1/1
  Constant8/1 -> GreaterThan1/2
  GreaterThan1/1 -> Switch5/2
  [right_lane_obstacles] -> Switch5/1
  [last_vaild_objDistY] -> Plus/1, Display4/1
  MRR_ObjDistY/1 -> [MRR_ObjDistY]
  [MRR_ObjDistY] -> Product/2
  MRR_ObjRelVelY/1 -> [MRR_ObjRelVelY]
  [MRR_ObjDistY] -> Product1/2
